simulink library "PCMULib"  (R2022b)
settings: Solver=ode45  StartTime=0.0  StopTime=10.0  RelTol=1e-3  EnableMultiTasking=on
undefined symbols (not defined in the file or in its folder): BreakpointData, BreakpointData1, BreakpointData2, BreakpointData_One_A, BreakpointData_Two_A, caaaa_dbi, caaaa_swi, cTmComprCtrl_n_i16SM4CmpHeatKiMax, cTmComprCtrl_n_i16SM4CmpHeatKiMin, cTmComprCtrl_n_i16SM4CmpHeatKpMax, cTmComprCtrl_n_i16SM4CmpHeatKpMin, cTmComprCtrl_Te_s32ErrCmpPIContinueHeatH, cTmComprCtrl_Te_s32ErrCmpPIContinueHeatL, cTmIn_n_ElacCmprReq_db, cTmIn_n_ElacCmprReq_sw, db, dbi, E2E_P01DataIDMode, E2E_P01ReceiverStatusType, EnumClass, iBit, initalValue, No_Runnable_Period, ObB_EidBsgStDerat_C, p_OVERRIDE_MASTER_SWITCH, SlDemoSign, sw, swi, SwitchOff_P, SwitchOn_P, Table, TableData_M, VCCTi33, VSysD_FidVehDerat1_C
libraries: simulink x22, CCMLib x11, simulink_need_slupdate x9, UXFD_Lib x7, canmsglib x2, PTCC_Lib x1, hdlsllib x1
(part 6 of 7)

== system PCMULib/Standard/Discrete dynamics/LPF1_discreteReset ==
  u : Inport
  a : Inport  Port=2
  r : Inport  Port=3
  LogicalSwitch1 : Subsystem  mask(PAG_Switch_LV1.6_BV2){}
      mask help:
      | Pass through input 1 when input 3 is true;
      | otherwise, pass through input 2
      mask Display:
      | plot([-0.1 0.2 0.2], [0.85 0.85 0.75])
      | plot([-0.1 0.2 0.2], [0.5 0.5 0.6])
      | plot([0.8 1.1], [0.5 0.5])
      | plot([0.15 0.8], [0.6 0.5])
      | plot([-0.1 0.5 0.5], [0.15 0.15 0.6])
  Product : Product  InputSameDT=on  RndMeth=Zero  SaturateOnIntegerOverflow=on  OutDataTypeStr=Inherit: Same as first input  mask(TL_Product){data={'logdata',{'maxnumvals',4096,'plotchannels',[]},'output',{'type','Float32'},'date',735300.29228090274}}
      settings: CopyFcn=if exist('tl_reset_reviewflag','file')==2,tl_reset_reviewflag(gcbh);end  DeleteFcn=if exist('delete_tlblock','file')==2,delete_tlblock(gcbh);end  NameChangeFcn=if exist('rename_tlblock','file')==2,rename_tlblock(gcbh);end  OpenFcn=if exist('tl_open_blockdlg','file')==2,tl_open_blockdlg(gcbh);else,open_system(gcbh,'parameter');end
      mask Help: eval(['if exist(''tl_online_help'',''file'') == 2, tl_online_help(''Topic'',''TL_Product''),else, web([''jar:file:///'',matlabroot,''/help/toolbox/simulink/help.jar!/slref/' lower(get_param(gcbh,'Blocktype')) '.html''], ''-helpbrowser''),end'])
      mask Display: plot([-0.05, 1.05, NaN, -0.05, 1.05],[.01, .01, NaN, .99, .99])
  Sum : Sum  Inputs=+-  InputSameDT=on  SaturateOnIntegerOverflow=on  OutDataTypeStr=Inherit: Same as first input  mask(TL_Sum){data={'logdata',{'maxnumvals',4096,'plotchannels',[]},'output',{'type','Float32'},'date',735300.29228062497}}
      settings: CopyFcn=if exist('tl_reset_reviewflag','file')==2,tl_reset_reviewflag(gcbh);end  DeleteFcn=if exist('delete_tlblock','file')==2,delete_tlblock(gcbh);end  NameChangeFcn=if exist('rename_tlblock','file')==2,rename_tlblock(gcbh);end  OpenFcn=if exist('tl_open_blockdlg','file')==2,tl_open_blockdlg(gcbh);else,open_system(gcbh,'parameter');end
      mask Help: eval(['if exist(''tl_online_help'',''file'') == 2, tl_online_help(''Topic'',''TL_Sum''),else, web([''jar:file:///'',matlabroot,''/help/toolbox/simulink/help.jar!/slref/' lower(get_param(gcbh,'Blocktype')) '.html''], ''-helpbrowser''),end'])
      mask Display: plot([-0.05, 1.05, NaN, -0.05, 1.05],[.01, .01, NaN, .99, .99])
  Sum1 : Sum  InputSameDT=on  SaturateOnIntegerOverflow=on  OutDataTypeStr=Inherit: Same as first input  mask(TL_Sum){data={'logdata',{'maxnumvals',4096,'plotchannels',[]},'output',{'type','Float32'},'date',735300.2922803472}}
      settings: CopyFcn=if exist('tl_reset_reviewflag','file')==2,tl_reset_reviewflag(gcbh);end  DeleteFcn=if exist('delete_tlblock','file')==2,delete_tlblock(gcbh);end  NameChangeFcn=if exist('rename_tlblock','file')==2,rename_tlblock(gcbh);end  OpenFcn=if exist('tl_open_blockdlg','file')==2,tl_open_blockdlg(gcbh);else,open_system(gcbh,'parameter');end
      mask Help: eval(['if exist(''tl_online_help'',''file'') == 2, tl_online_help(''Topic'',''TL_Sum''),else, web([''jar:file:///'',matlabroot,''/help/toolbox/simulink/help.jar!/slref/' lower(get_param(gcbh,'Blocktype')) '.html''], ''-helpbrowser''),end'])
      mask Display: plot([-0.05, 1.05, NaN, -0.05, 1.05],[.01, .01, NaN, .99, .99])
  UnitDelay : UnitDelay  SampleTime=-1  HasFrameUpgradeWarning=on  mask(TL_UnitDelay){data={'logdata',{'maxnumvals',4096,'plotchannels',[]},'output',{'type','Float32'},'state',{'type','Float32'},'date',735300.29228006944}}
      settings: CopyFcn=if exist('tl_reset_reviewflag','file')==2,tl_reset_reviewflag(gcbh);end  DeleteFcn=if exist('delete_tlblock','file')==2,delete_tlblock(gcbh);end  NameChangeFcn=if exist('rename_tlblock','file')==2,rename_tlblock(gcbh);end  OpenFcn=if exist('tl_open_blockdlg','file')==2,tl_open_blockdlg(gcbh);else,open_system(gcbh,'parameter');end
      mask Help: eval(['if exist(''tl_online_help'',''file'') == 2, tl_online_help(''Topic'',''TL_UnitDelay''),else, web([''jar:file:///'',matlabroot,''/help/toolbox/simulink/help.jar!/slref/' lower(get_param(gcbh,'Blocktype')) '.html''], ''-helpbrowser''),end'])
      mask Display: plot([-0.05, 1.05, NaN, -0.05, 1.05],[.01, .01, NaN, .99, .99])
  y : Outport
  wires:
  Product/1 -> Sum1/1
  a/1 -> Product/2
  Sum/1 -> Product/1
  u/1 -> Sum/2, Sum1/2, LogicalSwitch1/1(In1)
  r/1 -> LogicalSwitch1/3(In2)
  UnitDelay/1 -> Sum/1
  Sum1/1 -> LogicalSwitch1/2(In3)
  LogicalSwitch1/1(Out1) -> y/1, UnitDelay/1

== system PCMULib/Standard/Discrete dynamics/LPF2_discrete ==
  u : Inport
  a1 : Inport  Port=2
  a2 : Inport  Port=3
  b0 : Inport  Port=4
  b1 : Inport  Port=5
  b2 : Inport  Port=6
  Product : Product  InputSameDT=on  RndMeth=Zero  SaturateOnIntegerOverflow=on  OutDataTypeStr=Inherit: Same as first input  mask(TL_Product){data={'logdata',{'maxnumvals',4096,'plotchannels',[]},'output',{'type','Float32'},'date',735300.29227971064}}
      settings: CopyFcn=if exist('tl_reset_reviewflag','file')==2,tl_reset_reviewflag(gcbh);end  DeleteFcn=if exist('delete_tlblock','file')==2,delete_tlblock(gcbh);end  NameChangeFcn=if exist('rename_tlblock','file')==2,rename_tlblock(gcbh);end  OpenFcn=if exist('tl_open_blockdlg','file')==2,tl_open_blockdlg(gcbh);else,open_system(gcbh,'parameter');end
      mask Help: eval(['if exist(''tl_online_help'',''file'') == 2, tl_online_help(''Topic'',''TL_Product''),else, web([''jar:file:///'',matlabroot,''/help/toolbox/simulink/help.jar!/slref/' lower(get_param(gcbh,'Blocktype')) '.html''], ''-helpbrowser''),end'])
      mask Display: plot([-0.05, 1.05, NaN, -0.05, 1.05],[.01, .01, NaN, .99, .99])
  Product1 : Product  InputSameDT=on  RndMeth=Zero  SaturateOnIntegerOverflow=on  OutDataTypeStr=Inherit: Same as first input  mask(TL_Product){data={'logdata',{'maxnumvals',4096,'plotchannels',[]},'output',{'type','Float32'},'date',735300.29227943288}}
      settings: CopyFcn=if exist('tl_reset_reviewflag','file')==2,tl_reset_reviewflag(gcbh);end  DeleteFcn=if exist('delete_tlblock','file')==2,delete_tlblock(gcbh);end  NameChangeFcn=if exist('rename_tlblock','file')==2,rename_tlblock(gcbh);end  OpenFcn=if exist('tl_open_blockdlg','file')==2,tl_open_blockdlg(gcbh);else,open_system(gcbh,'parameter');end
      mask Help: eval(['if exist(''tl_online_help'',''file'') == 2, tl_online_help(''Topic'',''TL_Product''),else, web([''jar:file:///'',matlabroot,''/help/toolbox/simulink/help.jar!/slref/' lower(get_param(gcbh,'Blocktype')) '.html''], ''-helpbrowser''),end'])
      mask Display: plot([-0.05, 1.05, NaN, -0.05, 1.05],[.01, .01, NaN, .99, .99])
  Product2 : Product  InputSameDT=on  RndMeth=Zero  SaturateOnIntegerOverflow=on  OutDataTypeStr=Inherit: Same as first input  mask(TL_Product){data={'logdata',{'maxnumvals',4096,'plotchannels',[]},'output',{'type','Float32'},'date',735300.29227915511}}
      settings: CopyFcn=if exist('tl_reset_reviewflag','file')==2,tl_reset_reviewflag(gcbh);end  DeleteFcn=if exist('delete_tlblock','file')==2,delete_tlblock(gcbh);end  NameChangeFcn=if exist('rename_tlblock','file')==2,rename_tlblock(gcbh);end  OpenFcn=if exist('tl_open_blockdlg','file')==2,tl_open_blockdlg(gcbh);else,open_system(gcbh,'parameter');end
      mask Help: eval(['if exist(''tl_online_help'',''file'') == 2, tl_online_help(''Topic'',''TL_Product''),else, web([''jar:file:///'',matlabroot,''/help/toolbox/simulink/help.jar!/slref/' lower(get_param(gcbh,'Blocktype')) '.html''], ''-helpbrowser''),end'])
      mask Display: plot([-0.05, 1.05, NaN, -0.05, 1.05],[.01, .01, NaN, .99, .99])
  Product3 : Product  InputSameDT=on  RndMeth=Zero  SaturateOnIntegerOverflow=on  OutDataTypeStr=Inherit: Same as first input  mask(TL_Product){data={'logdata',{'maxnumvals',4096,'plotchannels',[]},'output',{'type','Float32'},'date',735300.29227888887}}
      settings: CopyFcn=if exist('tl_reset_reviewflag','file')==2,tl_reset_reviewflag(gcbh);end  DeleteFcn=if exist('delete_tlblock','file')==2,delete_tlblock(gcbh);end  NameChangeFcn=if exist('rename_tlblock','file')==2,rename_tlblock(gcbh);end  OpenFcn=if exist('tl_open_blockdlg','file')==2,tl_open_blockdlg(gcbh);else,open_system(gcbh,'parameter');end
      mask Help: eval(['if exist(''tl_online_help'',''file'') == 2, tl_online_help(''Topic'',''TL_Product''),else, web([''jar:file:///'',matlabroot,''/help/toolbox/simulink/help.jar!/slref/' lower(get_param(gcbh,'Blocktype')) '.html''], ''-helpbrowser''),end'])
      mask Display: plot([-0.05, 1.05, NaN, -0.05, 1.05],[.01, .01, NaN, .99, .99])
  Product4 : Product  InputSameDT=on  RndMeth=Zero  SaturateOnIntegerOverflow=on  OutDataTypeStr=Inherit: Same as first input  mask(TL_Product){data={'logdata',{'maxnumvals',4096,'plotchannels',[]},'output',{'type','Float32'},'date',735300.2922786111}}
      settings: CopyFcn=if exist('tl_reset_reviewflag','file')==2,tl_reset_reviewflag(gcbh);end  DeleteFcn=if exist('delete_tlblock','file')==2,delete_tlblock(gcbh);end  NameChangeFcn=if exist('rename_tlblock','file')==2,rename_tlblock(gcbh);end  OpenFcn=if exist('tl_open_blockdlg','file')==2,tl_open_blockdlg(gcbh);else,open_system(gcbh,'parameter');end
      mask Help: eval(['if exist(''tl_online_help'',''file'') == 2, tl_online_help(''Topic'',''TL_Product''),else, web([''jar:file:///'',matlabroot,''/help/toolbox/simulink/help.jar!/slref/' lower(get_param(gcbh,'Blocktype')) '.html''], ''-helpbrowser''),end'])
      mask Display: plot([-0.05, 1.05, NaN, -0.05, 1.05],[.01, .01, NaN, .99, .99])
  Sum : Sum  Inputs=+++--  InputSameDT=on  SaturateOnIntegerOverflow=on  OutDataTypeStr=Inherit: Same as first input  mask(TL_Sum){data={'logdata',{'maxnumvals',4096,'plotchannels',[]},'output',{'type','Float32'},'date',735300.29227833333}}
      settings: CopyFcn=if exist('tl_reset_reviewflag','file')==2,tl_reset_reviewflag(gcbh);end  DeleteFcn=if exist('delete_tlblock','file')==2,delete_tlblock(gcbh);end  NameChangeFcn=if exist('rename_tlblock','file')==2,rename_tlblock(gcbh);end  OpenFcn=if exist('tl_open_blockdlg','file')==2,tl_open_blockdlg(gcbh);else,open_system(gcbh,'parameter');end
      mask Help: eval(['if exist(''tl_online_help'',''file'') == 2, tl_online_help(''Topic'',''TL_Sum''),else, web([''jar:file:///'',matlabroot,''/help/toolbox/simulink/help.jar!/slref/' lower(get_param(gcbh,'Blocktype')) '.html''], ''-helpbrowser''),end'])
      mask Display: plot([-0.05, 1.05, NaN, -0.05, 1.05],[.01, .01, NaN, .99, .99])
  UnitDelay : UnitDelay  SampleTime=-1  HasFrameUpgradeWarning=on  mask(TL_UnitDelay){data={'logdata',{'maxnumvals',4096,'plotchannels',[]},'output',{'type','Float32'},'state',{'type','Float32'},'date',735300.29227804393}}
      settings: CopyFcn=if exist('tl_reset_reviewflag','file')==2,tl_reset_reviewflag(gcbh);end  DeleteFcn=if exist('delete_tlblock','file')==2,delete_tlblock(gcbh);end  NameChangeFcn=if exist('rename_tlblock','file')==2,rename_tlblock(gcbh);end  OpenFcn=if exist('tl_open_blockdlg','file')==2,tl_open_blockdlg(gcbh);else,open_system(gcbh,'parameter');end
      mask Help: eval(['if exist(''tl_online_help'',''file'') == 2, tl_online_help(''Topic'',''TL_UnitDelay''),else, web([''jar:file:///'',matlabroot,''/help/toolbox/simulink/help.jar!/slref/' lower(get_param(gcbh,'Blocktype')) '.html''], ''-helpbrowser''),end'])
      mask Display: plot([-0.05, 1.05, NaN, -0.05, 1.05],[.01, .01, NaN, .99, .99])
  UnitDelay1 : UnitDelay  SampleTime=-1  HasFrameUpgradeWarning=on  mask(TL_UnitDelay){data={'logdata',{'maxnumvals',4096,'plotchannels',[]},'output',{'type','Float32'},'state',{'type','Float32'},'date',735300.29227769678}}
      settings: CopyFcn=if exist('tl_reset_reviewflag','file')==2,tl_reset_reviewflag(gcbh);end  DeleteFcn=if exist('delete_tlblock','file')==2,delete_tlblock(gcbh);end  NameChangeFcn=if exist('rename_tlblock','file')==2,rename_tlblock(gcbh);end  OpenFcn=if exist('tl_open_blockdlg','file')==2,tl_open_blockdlg(gcbh);else,open_system(gcbh,'parameter');end
      mask Help: eval(['if exist(''tl_online_help'',''file'') == 2, tl_online_help(''Topic'',''TL_UnitDelay''),else, web([''jar:file:///'',matlabroot,''/help/toolbox/simulink/help.jar!/slref/' lower(get_param(gcbh,'Blocktype')) '.html''], ''-helpbrowser''),end'])
      mask Display: plot([-0.05, 1.05, NaN, -0.05, 1.05],[.01, .01, NaN, .99, .99])
  UnitDelay2 : UnitDelay  SampleTime=-1  HasFrameUpgradeWarning=on  mask(TL_UnitDelay){data={'logdata',{'maxnumvals',4096,'plotchannels',[]},'output',{'type','Float32'},'state',{'type','Float32'},'date',735300.29227733798}}
      settings: CopyFcn=if exist('tl_reset_reviewflag','file')==2,tl_reset_reviewflag(gcbh);end  DeleteFcn=if exist('delete_tlblock','file')==2,delete_tlblock(gcbh);end  NameChangeFcn=if exist('rename_tlblock','file')==2,rename_tlblock(gcbh);end  OpenFcn=if exist('tl_open_blockdlg','file')==2,tl_open_blockdlg(gcbh);else,open_system(gcbh,'parameter');end
      mask Help: eval(['if exist(''tl_online_help'',''file'') == 2, tl_online_help(''Topic'',''TL_UnitDelay''),else, web([''jar:file:///'',matlabroot,''/help/toolbox/simulink/help.jar!/slref/' lower(get_param(gcbh,'Blocktype')) '.html''], ''-helpbrowser''),end'])
      mask Display: plot([-0.05, 1.05, NaN, -0.05, 1.05],[.01, .01, NaN, .99, .99])
  UnitDelay3 : UnitDelay  SampleTime=-1  HasFrameUpgradeWarning=on  mask(TL_UnitDelay){data={'logdata',{'maxnumvals',4096,'plotchannels',[]},'output',{'type','Float32'},'state',{'type','Float32'},'date',735300.29227697919}}
      settings: CopyFcn=if exist('tl_reset_reviewflag','file')==2,tl_reset_reviewflag(gcbh);end  DeleteFcn=if exist('delete_tlblock','file')==2,delete_tlblock(gcbh);end  NameChangeFcn=if exist('rename_tlblock','file')==2,rename_tlblock(gcbh);end  OpenFcn=if exist('tl_open_blockdlg','file')==2,tl_open_blockdlg(gcbh);else,open_system(gcbh,'parameter');end
      mask Help: eval(['if exist(''tl_online_help'',''file'') == 2, tl_online_help(''Topic'',''TL_UnitDelay''),else, web([''jar:file:///'',matlabroot,''/help/toolbox/simulink/help.jar!/slref/' lower(get_param(gcbh,'Blocktype')) '.html''], ''-helpbrowser''),end'])
      mask Display: plot([-0.05, 1.05, NaN, -0.05, 1.05],[.01, .01, NaN, .99, .99])
  y : Outport
  wires:
  UnitDelay3/1 -> Product4/2
  Product2/1 -> Sum/1
  Product1/1 -> Sum/2
  UnitDelay2/1 -> Product2/1
  b2/1 -> Product2/2
  b1/1 -> Product1/2
  Product/1 -> Sum/3
  Product3/1 -> Sum/4
  a1/1 -> Product3/1
  b0/1 -> Product/2
  a2/1 -> Product4/1
  Product4/1 -> Sum/5
  UnitDelay/1 -> UnitDelay2/1, Product1/1
  u/1 -> UnitDelay/1, Product/1
  Sum/1 -> y/1, UnitDelay1/1
  UnitDelay1/1 -> Product3/2, UnitDelay3/1

== system PCMULib/Standard/Discrete dynamics/LPF2_omega ==
  u : Inport
  w : Inport  Port=2
  z : Inport  Port=3
  Constant : Constant  Value=2  mask(TL_Constant){data={'output',{'type','Float32'},'date',735300.29222866893}}
      settings: CopyFcn=if exist('tl_reset_reviewflag','file')==2,tl_reset_reviewflag(gcbh);end  DeleteFcn=if exist('delete_tlblock','file')==2,delete_tlblock(gcbh);end  NameChangeFcn=if exist('rename_tlblock','file')==2,rename_tlblock(gcbh);end  OpenFcn=if exist('tl_open_blockdlg','file')==2,tl_open_blockdlg(gcbh);else,open_system(gcbh,'parameter');end
      mask Help: eval(['if exist(''tl_online_help'',''file'') == 2, tl_online_help(''Topic'',''TL_Constant''),else, web([''jar:file:///'',matlabroot,''/help/toolbox/simulink/help.jar!/slref/' lower(get_param(gcbh,'Blocktype')) '.html''], ''-helpbrowser''),end'])
      mask Display: plot([-0.05, 1.05, NaN, -0.05, 1.05],[.01, .01, NaN, .99, .99])
  Constant2 : Constant  Value=2  mask(TL_Constant){data={'output',{'type','Float32'},'date',735300.29222841433}}
      settings: CopyFcn=if exist('tl_reset_reviewflag','file')==2,tl_reset_reviewflag(gcbh);end  DeleteFcn=if exist('delete_tlblock','file')==2,delete_tlblock(gcbh);end  NameChangeFcn=if exist('rename_tlblock','file')==2,rename_tlblock(gcbh);end  OpenFcn=if exist('tl_open_blockdlg','file')==2,tl_open_blockdlg(gcbh);else,open_system(gcbh,'parameter');end
      mask Help: eval(['if exist(''tl_online_help'',''file'') == 2, tl_online_help(''Topic'',''TL_Constant''),else, web([''jar:file:///'',matlabroot,''/help/toolbox/simulink/help.jar!/slref/' lower(get_param(gcbh,'Blocktype')) '.html''], ''-helpbrowser''),end'])
      mask Display: plot([-0.05, 1.05, NaN, -0.05, 1.05],[.01, .01, NaN, .99, .99])
  Constant3 : Constant  mask(TL_Constant){data={'output',{'type','Float32'},'date',735300.29222815973}}
      settings: CopyFcn=if exist('tl_reset_reviewflag','file')==2,tl_reset_reviewflag(gcbh);end  DeleteFcn=if exist('delete_tlblock','file')==2,delete_tlblock(gcbh);end  NameChangeFcn=if exist('rename_tlblock','file')==2,rename_tlblock(gcbh);end  OpenFcn=if exist('tl_open_blockdlg','file')==2,tl_open_blockdlg(gcbh);else,open_system(gcbh,'parameter');end
      mask Help: eval(['if exist(''tl_online_help'',''file'') == 2, tl_online_help(''Topic'',''TL_Constant''),else, web([''jar:file:///'',matlabroot,''/help/toolbox/simulink/help.jar!/slref/' lower(get_param(gcbh,'Blocktype')) '.html''], ''-helpbrowser''),end'])
      mask Display: plot([-0.05, 1.05, NaN, -0.05, 1.05],[.01, .01, NaN, .99, .99])
  Product : Product  Inputs=**  InputSameDT=on  RndMeth=Zero  SaturateOnIntegerOverflow=on  OutDataTypeStr=Inherit: Same as first input  mask(TL_Product){data={'logdata',{'maxnumvals',4096,'plotchannels',[]},'output',{'type','Float32'},'date',735300.29222787032}}
      settings: CopyFcn=if exist('tl_reset_reviewflag','file')==2,tl_reset_reviewflag(gcbh);end  DeleteFcn=if exist('delete_tlblock','file')==2,delete_tlblock(gcbh);end  NameChangeFcn=if exist('rename_tlblock','file')==2,rename_tlblock(gcbh);end  OpenFcn=if exist('tl_open_blockdlg','file')==2,tl_open_blockdlg(gcbh);else,open_system(gcbh,'parameter');end
      mask Help: eval(['if exist(''tl_online_help'',''file'') == 2, tl_online_help(''Topic'',''TL_Product''),else, web([''jar:file:///'',matlabroot,''/help/toolbox/simulink/help.jar!/slref/' lower(get_param(gcbh,'Blocktype')) '.html''], ''-helpbrowser''),end'])
      mask Display: plot([-0.05, 1.05, NaN, -0.05, 1.05],[.01, .01, NaN, .99, .99])
  Product1 : Product  Inputs=***  InputSameDT=on  RndMeth=Zero  SaturateOnIntegerOverflow=on  OutDataTypeStr=Inherit: Same as first input  mask(TL_Product){data={'logdata',{'maxnumvals',4096,'plotchannels',[]},'output',{'type','Float32'},'date',735300.29222759255}}
      settings: CopyFcn=if exist('tl_reset_reviewflag','file')==2,tl_reset_reviewflag(gcbh);end  DeleteFcn=if exist('delete_tlblock','file')==2,delete_tlblock(gcbh);end  NameChangeFcn=if exist('rename_tlblock','file')==2,rename_tlblock(gcbh);end  OpenFcn=if exist('tl_open_blockdlg','file')==2,tl_open_blockdlg(gcbh);else,open_system(gcbh,'parameter');end
      mask Help: eval(['if exist(''tl_online_help'',''file'') == 2, tl_online_help(''Topic'',''TL_Product''),else, web([''jar:file:///'',matlabroot,''/help/toolbox/simulink/help.jar!/slref/' lower(get_param(gcbh,'Blocktype')) '.html''], ''-helpbrowser''),end'])
      mask Display: plot([-0.05, 1.05, NaN, -0.05, 1.05],[.01, .01, NaN, .99, .99])
  Product3 : Product  Inputs=**  InputSameDT=on  RndMeth=Zero  SaturateOnIntegerOverflow=on  OutDataTypeStr=Inherit: Same as first input  mask(TL_Product){data={'logdata',{'maxnumvals',4096,'plotchannels',[]},'output',{'type','Float32'},'date',735300.29222732643}}
      settings: CopyFcn=if exist('tl_reset_reviewflag','file')==2,tl_reset_reviewflag(gcbh);end  DeleteFcn=if exist('delete_tlblock','file')==2,delete_tlblock(gcbh);end  NameChangeFcn=if exist('rename_tlblock','file')==2,rename_tlblock(gcbh);end  OpenFcn=if exist('tl_open_blockdlg','file')==2,tl_open_blockdlg(gcbh);else,open_system(gcbh,'parameter');end
      mask Help: eval(['if exist(''tl_online_help'',''file'') == 2, tl_online_help(''Topic'',''TL_Product''),else, web([''jar:file:///'',matlabroot,''/help/toolbox/simulink/help.jar!/slref/' lower(get_param(gcbh,'Blocktype')) '.html''], ''-helpbrowser''),end'])
      mask Display: plot([-0.05, 1.05, NaN, -0.05, 1.05],[.01, .01, NaN, .99, .99])
  Product4 : Product  Inputs=**  InputSameDT=on  RndMeth=Zero  SaturateOnIntegerOverflow=on  OutDataTypeStr=Inherit: Same as first input  mask(TL_Product){data={'logdata',{'maxnumvals',4096,'plotchannels',[]},'output',{'type','Float32'},'date',735300.29222704866}}
      settings: CopyFcn=if exist('tl_reset_reviewflag','file')==2,tl_reset_reviewflag(gcbh);end  DeleteFcn=if exist('delete_tlblock','file')==2,delete_tlblock(gcbh);end  NameChangeFcn=if exist('rename_tlblock','file')==2,rename_tlblock(gcbh);end  OpenFcn=if exist('tl_open_blockdlg','file')==2,tl_open_blockdlg(gcbh);else,open_system(gcbh,'parameter');end
      mask Help: eval(['if exist(''tl_online_help'',''file'') == 2, tl_online_help(''Topic'',''TL_Product''),else, web([''jar:file:///'',matlabroot,''/help/toolbox/simulink/help.jar!/slref/' lower(get_param(gcbh,'Blocktype')) '.html''], ''-helpbrowser''),end'])
      mask Display: plot([-0.05, 1.05, NaN, -0.05, 1.05],[.01, .01, NaN, .99, .99])
  Product5 : Product  Inputs=*/  InputSameDT=on  RndMeth=Zero  SaturateOnIntegerOverflow=on  OutDataTypeStr=Inherit: Same as first input  mask(TL_Product){data={'logdata',{'maxnumvals',4096,'plotchannels',[]},'output',{'type','Float32'},'date',735300.29222677078}}
      settings: CopyFcn=if exist('tl_reset_reviewflag','file')==2,tl_reset_reviewflag(gcbh);end  DeleteFcn=if exist('delete_tlblock','file')==2,delete_tlblock(gcbh);end  NameChangeFcn=if exist('rename_tlblock','file')==2,rename_tlblock(gcbh);end  OpenFcn=if exist('tl_open_blockdlg','file')==2,tl_open_blockdlg(gcbh);else,open_system(gcbh,'parameter');end
      mask Help: eval(['if exist(''tl_online_help'',''file'') == 2, tl_online_help(''Topic'',''TL_Product''),else, web([''jar:file:///'',matlabroot,''/help/toolbox/simulink/help.jar!/slref/' lower(get_param(gcbh,'Blocktype')) '.html''], ''-helpbrowser''),end'])
      mask Display: plot([-0.05, 1.05, NaN, -0.05, 1.05],[.01, .01, NaN, .99, .99])
  Product6 : Product  Inputs=**  InputSameDT=on  RndMeth=Zero  SaturateOnIntegerOverflow=on  OutDataTypeStr=Inherit: Same as first input  mask(TL_Product){data={'logdata',{'maxnumvals',4096,'plotchannels',[]},'output',{'type','Float32'},'date',735300.29222649301}}
      settings: CopyFcn=if exist('tl_reset_reviewflag','file')==2,tl_reset_reviewflag(gcbh);end  DeleteFcn=if exist('delete_tlblock','file')==2,delete_tlblock(gcbh);end  NameChangeFcn=if exist('rename_tlblock','file')==2,rename_tlblock(gcbh);end  OpenFcn=if exist('tl_open_blockdlg','file')==2,tl_open_blockdlg(gcbh);else,open_system(gcbh,'parameter');end
      mask Help: eval(['if exist(''tl_online_help'',''file'') == 2, tl_online_help(''Topic'',''TL_Product''),else, web([''jar:file:///'',matlabroot,''/help/toolbox/simulink/help.jar!/slref/' lower(get_param(gcbh,'Blocktype')) '.html''], ''-helpbrowser''),end'])
      mask Display: plot([-0.05, 1.05, NaN, -0.05, 1.05],[.01, .01, NaN, .99, .99])
  Sum1 : Sum  Inputs=+--  InputSameDT=on  SaturateOnIntegerOverflow=on  OutDataTypeStr=Inherit: Same as first input  mask(TL_Sum){data={'logdata',{'maxnumvals',4096,'plotchannels',[]},'output',{'type','Float32'},'date',735300.29222619208}}
      settings: CopyFcn=if exist('tl_reset_reviewflag','file')==2,tl_reset_reviewflag(gcbh);end  DeleteFcn=if exist('delete_tlblock','file')==2,delete_tlblock(gcbh);end  NameChangeFcn=if exist('rename_tlblock','file')==2,rename_tlblock(gcbh);end  OpenFcn=if exist('tl_open_blockdlg','file')==2,tl_open_blockdlg(gcbh);else,open_system(gcbh,'parameter');end
      mask Help: eval(['if exist(''tl_online_help'',''file'') == 2, tl_online_help(''Topic'',''TL_Sum''),else, web([''jar:file:///'',matlabroot,''/help/toolbox/simulink/help.jar!/slref/' lower(get_param(gcbh,'Blocktype')) '.html''], ''-helpbrowser''),end'])
      mask Display: plot([-0.05, 1.05, NaN, -0.05, 1.05],[.01, .01, NaN, .99, .99])
  Sum2 : Sum  Inputs=--  InputSameDT=on  SaturateOnIntegerOverflow=on  OutDataTypeStr=Inherit: Same as first input  mask(TL_Sum){data={'logdata',{'maxnumvals',4096,'plotchannels',[]},'output',{'type','Float32'},'date',735300.29222592595}}
      settings: CopyFcn=if exist('tl_reset_reviewflag','file')==2,tl_reset_reviewflag(gcbh);end  DeleteFcn=if exist('delete_tlblock','file')==2,delete_tlblock(gcbh);end  NameChangeFcn=if exist('rename_tlblock','file')==2,rename_tlblock(gcbh);end  OpenFcn=if exist('tl_open_blockdlg','file')==2,tl_open_blockdlg(gcbh);else,open_system(gcbh,'parameter');end
      mask Help: eval(['if exist(''tl_online_help'',''file'') == 2, tl_online_help(''Topic'',''TL_Sum''),else, web([''jar:file:///'',matlabroot,''/help/toolbox/simulink/help.jar!/slref/' lower(get_param(gcbh,'Blocktype')) '.html''], ''-helpbrowser''),end'])
      mask Display: plot([-0.05, 1.05, NaN, -0.05, 1.05],[.01, .01, NaN, .99, .99])
  Sum3 : Sum  Inputs=+++  InputSameDT=on  SaturateOnIntegerOverflow=on  OutDataTypeStr=Inherit: Same as first input  mask(TL_Sum){data={'logdata',{'maxnumvals',4096,'plotchannels',[]},'output',{'type','Float32'},'date',735300.29222564818}}
      settings: CopyFcn=if exist('tl_reset_reviewflag','file')==2,tl_reset_reviewflag(gcbh);end  DeleteFcn=if exist('delete_tlblock','file')==2,delete_tlblock(gcbh);end  NameChangeFcn=if exist('rename_tlblock','file')==2,rename_tlblock(gcbh);end  OpenFcn=if exist('tl_open_blockdlg','file')==2,tl_open_blockdlg(gcbh);else,open_system(gcbh,'parameter');end
      mask Help: eval(['if exist(''tl_online_help'',''file'') == 2, tl_online_help(''Topic'',''TL_Sum''),else, web([''jar:file:///'',matlabroot,''/help/toolbox/simulink/help.jar!/slref/' lower(get_param(gcbh,'Blocktype')) '.html''], ''-helpbrowser''),end'])
      mask Display: plot([-0.05, 1.05, NaN, -0.05, 1.05],[.01, .01, NaN, .99, .99])
  UnitDelay1 : UnitDelay  SampleTime=-1  HasFrameUpgradeWarning=on  mask(TL_UnitDelay){data={'logdata',{'maxnumvals',4096,'plotchannels',[]},'output',{'type','Float32'},'state',{'type','Float32'},'date',735300.29222532408}}
      settings: CopyFcn=if exist('tl_reset_reviewflag','file')==2,tl_reset_reviewflag(gcbh);end  DeleteFcn=if exist('delete_tlblock','file')==2,delete_tlblock(gcbh);end  NameChangeFcn=if exist('rename_tlblock','file')==2,rename_tlblock(gcbh);end  OpenFcn=if exist('tl_open_blockdlg','file')==2,tl_open_blockdlg(gcbh);else,open_system(gcbh,'parameter');end
      mask Help: eval(['if exist(''tl_online_help'',''file'') == 2, tl_online_help(''Topic'',''TL_UnitDelay''),else, web([''jar:file:///'',matlabroot,''/help/toolbox/simulink/help.jar!/slref/' lower(get_param(gcbh,'Blocktype')) '.html''], ''-helpbrowser''),end'])
      mask Display: plot([-0.05, 1.05, NaN, -0.05, 1.05],[.01, .01, NaN, .99, .99])
  UnitDelay3 : UnitDelay  SampleTime=-1  HasFrameUpgradeWarning=on  mask(TL_UnitDelay){data={'logdata',{'maxnumvals',4096,'plotchannels',[]},'output',{'type','Float32'},'state',{'type','Float32'},'date',735300.29222478007}}
      settings: CopyFcn=if exist('tl_reset_reviewflag','file')==2,tl_reset_reviewflag(gcbh);end  DeleteFcn=if exist('delete_tlblock','file')==2,delete_tlblock(gcbh);end  NameChangeFcn=if exist('rename_tlblock','file')==2,rename_tlblock(gcbh);end  OpenFcn=if exist('tl_open_blockdlg','file')==2,tl_open_blockdlg(gcbh);else,open_system(gcbh,'parameter');end
      mask Help: eval(['if exist(''tl_online_help'',''file'') == 2, tl_online_help(''Topic'',''TL_UnitDelay''),else, web([''jar:file:///'',matlabroot,''/help/toolbox/simulink/help.jar!/slref/' lower(get_param(gcbh,'Blocktype')) '.html''], ''-helpbrowser''),end'])
      mask Display: plot([-0.05, 1.05, NaN, -0.05, 1.05],[.01, .01, NaN, .99, .99])
  ts : DataStoreRead  DataStoreName=ts  IndexOptions=Index vector (dialog)  Indices=1  OutputSizes=1  mask(TL_DataStoreRead){data={'logdata',{'plotchannels',[]},'date',735300.29222303245}}
      settings: AttributesFormatString=ts  DeleteFcn=if exist('delete_tlblock','file')==2,delete_tlblock(gcbh);end  NameChangeFcn=if exist('rename_tlblock','file')==2,rename_tlblock(gcbh);end  OpenFcn=if exist('tl_open_blockdlg','file')==2,tl_open_blockdlg(gcbh);else,open_system(gcbh,'parameter');end
      mask Help: eval(['if exist(''tl_online_help'',''file'') == 2, tl_online_help(''Topic'',''TL_DataStoreRead''),else, web([''jar:file:///'',matlabroot,''/help/toolbox/simulink/help.jar!/slref/' lower(get_param(gcbh,'Blocktype')) '.html''], ''-helpbrowser''),end'])
      mask Display: plot([-0.05, 1.05, NaN, -0.05, 1.05],[.01, .01, NaN, .99, .99])
  y : Outport
  wires:
  z/1 -> Product1/2
  UnitDelay3/1 -> Sum1/3
  Product3/1 -> Product6/2, Sum3/2
  Sum3/1 -> Product5/2
  Constant3/1 -> Sum3/3
  Product5/1 -> y/1, UnitDelay1/1
  Constant2/1 -> Sum2/1
  u/1 -> Product6/1
  Product6/1 -> Sum1/1
  Product4/1 -> Sum1/2
  Sum1/1 -> Product5/1
  Sum2/1 -> Product4/1
  ts/1 -> Product/2
  w/1 -> Product/1
  Constant/1 -> Product1/3
  Product1/1 -> Sum3/1, Sum2/2
  UnitDelay1/1 -> Product4/2, UnitDelay3/1
  Product/1 -> Product1/1, Product3/2, Product3/1

== system PCMULib/Standard/Discrete dynamics/RateLimit ==
  u : Inport
  d : Inport  Port=2
  Add : Sum  Inputs=+-
  Add1 : Sum
  MinMax : MinMax  Function=max  Inputs=2
  MinMax1 : MinMax  Inputs=2
  Product : Product
  Product1 : Product
  Unit Delay : UnitDelay  SampleTime=-1  HasFrameUpgradeWarning=on
  ts : DataStoreRead  DataStoreName=ts  IndexOptions=Index vector (dialog)  Indices=1  OutputSizes=1
  y : Outport
  wires:
  d/1 -> Product/1, Product1/2
  Product/1 -> Add1/1
  ts/1 -> Product/2, Product1/1
  Product1/1 -> Add/2
  Add/1 -> MinMax/2
  MinMax/1 -> MinMax1/1
  Unit Delay/1 -> Add1/2, Add/1
  Add1/1 -> MinMax1/2
  u/1 -> MinMax/1
  MinMax1/1 -> y/1, Unit Delay/1

== system PCMULib/Standard/Discrete dynamics/RateLimit1 ==
  In1 : Inport
  r : Inport  Port=2
  dr : Inport  Port=3
  r1 : Inport  Port=4
  Abs : Abs  SaturateOnIntegerOverflow=off
  Add : Sum  Inputs=+-
  Add1 : Sum
  MinMax : MinMax  Function=max  Inputs=2
  MinMax1 : MinMax  Inputs=2
  Product : Product
  Product1 : Product
  Switch : Switch  Criteria=u2 > Threshold  SaturateOnIntegerOverflow=off  InputSameDT=off
  Unit Delay : UnitDelay  SampleTime=-1  HasFrameUpgradeWarning=on
  ts : DataStoreRead  DataStoreName=ts  IndexOptions=Index vector (dialog)  Indices=1  OutputSizes=1
  y : Outport
  wires:
  Abs/1 -> Add/2
  In1/1 -> Switch/1, MinMax/1
  Add1/1 -> MinMax1/2
  Unit Delay/1 -> Add1/2, Add/1
  MinMax/1 -> MinMax1/1
  Product1/1 -> Abs/1
  ts/1 -> Product1/1, Product/2
  Product/1 -> Add1/1
  dr/1 -> Product/1
  MinMax1/1 -> Switch/3
  r/1 -> Switch/2
  Switch/1 -> y/1, Unit Delay/1
  r1/1 -> Product1/2
  Add/1 -> MinMax/2

== system PCMULib/Standard/Discrete dynamics/xbackground1 ==

== system PCMULib/Standard/Discrete dynamics/xbackground2 ==

== system PCMULib/Standard/Discrete dynamics/xbackground3 ==

== system PCMULib/Standard/Discrete dynamics/xbackground4 ==

== system PCMULib/Standard/Discrete dynamics/xbackground5 ==

== system PCMULib/Standard/Discrete dynamics/xbackground6 ==

== system PCMULib/Standard/Discrete dynamics/xbackground7 ==

== system PCMULib/Standard/Math/AbsForBoschCompiler ==
  In1 : Inport
  Gain : Gain  Gain=-1  OutDataTypeStr=Inherit: Same as input  ParamDataTypeStr=Inherit: Same as input  mask(TL_Gain){data={'logdata',{'plotchannels',[]},'output',{'type','Float32','unit','-'},'date',735300.29225025466}}
      settings: CopyFcn=if exist('tl_reset_reviewflag','file')==2,tl_reset_reviewflag(gcbh);end  DeleteFcn=if exist('delete_tlblock','file')==2,delete_tlblock(gcbh);end  NameChangeFcn=if exist('rename_tlblock','file')==2,rename_tlblock(gcbh);end  OpenFcn=if exist('tl_open_blockdlg','file')==2,tl_open_blockdlg(gcbh);else,open_system(gcbh,'parameter');end
      mask Help: eval(['if exist(''tl_online_help'',''file'') == 2, tl_online_help(''Topic'',''TL_Gain''),else, web([''jar:file:///'',matlabroot,''/help/toolbox/simulink/help.jar!/slref/' lower(get_param(gcbh,'Blocktype')) '.html''], ''-helpbrowser''),end'])
      mask Display: plot([0, .9, 0],[.05, .5, .95])
  Switch1 : Switch  SaturateOnIntegerOverflow=off  InputSameDT=off  mask(TL_Switch){data={'logdata',{'plotchannels',[]},'output',{'name','r$N_$L','class','CVC_DISP32','type','Float32'},'date',737070.42928155093}}
      settings: CopyFcn=if exist('tl_reset_reviewflag','file')==2,tl_reset_reviewflag(gcbh);end  DeleteFcn=if exist('delete_tlblock','file')==2,delete_tlblock(gcbh);end  NameChangeFcn=if exist('rename_tlblock','file')==2,rename_tlblock(gcbh);end  OpenFcn=if exist('tl_open_blockdlg','file')==2,tl_open_blockdlg(gcbh);else,open_system(gcbh,'parameter');end
      mask Help: eval(['if exist(''tl_online_help'',''file'') == 2, tl_online_help(''Topic'',''TL_Switch''),else, web([''jar:file:///'',matlabroot,''/help/toolbox/simulink/help.jar!/slref/' lower(get_param(gcbh,'Blocktype')) '.html''], ''-helpbrowser''),end'])
      mask Display: plot([-0.05, 1.05, NaN, -0.05, 1.05],[.01, .01, NaN, .99, .99])
  Out1 : Outport
  wires:
  Gain/1 -> Switch1/3
  In1/1 -> Gain/1, Switch1/2, Switch1/1
  Switch1/1 -> Out1/1  "rt_DFT2RevArgAbs"

== system PCMULib/Standard/Math/Floor ==
  In1 : Inport
  Add : Sum  Inputs=+-
  Constant : Constant
  mod1 : Subsystem  mask(GL_Mod_1.0){}
      mask help: Signed remainder after division.
      mask Display: disp('mod')
  Out1 : Outport
  wires:
  Constant/1 -> mod1/2(In2)
  Add/1 -> Out1/1
  In1/1 -> mod1/1(In1), Add/1
  mod1/1(Out1) -> Add/2

== system PCMULib/Standard/Math/Interpolation ==
  In1 : Inport
  x1 : Inport  Port=2
  y1 : Inport  Port=3
  x2 : Inport  Port=4
  y2 : Inport  Port=5
  Add : Sum  Inputs=+-
  Add1 : Sum  Inputs=+-
  Add2 : Sum  Inputs=+-
  Add3 : Sum
  Constant : Constant
  One3 : Constant  Value=1e-6  OutDataTypeStr=single  mask(TL_Constant){data={'output',{'type','Float32'},'date',735300.29224869213}}
      settings: CopyFcn=if exist('tl_reset_reviewflag','file')==2,tl_reset_reviewflag(gcbh);end  DeleteFcn=if exist('delete_tlblock','file')==2,delete_tlblock(gcbh);end  NameChangeFcn=if exist('rename_tlblock','file')==2,rename_tlblock(gcbh);end  OpenFcn=if exist('tl_open_blockdlg','file')==2,tl_open_blockdlg(gcbh);else,open_system(gcbh,'parameter');end
      mask Help: eval(['if exist(''tl_online_help'',''file'') == 2, tl_online_help(''Topic'',''TL_Constant''),else, web([''jar:file:///'',matlabroot,''/help/toolbox/simulink/help.jar!/slref/' lower(get_param(gcbh,'Blocktype')) '.html''], ''-helpbrowser''),end'])
      mask Display: plot([-0.05, 1.05, NaN, -0.05, 1.05],[.01, .01, NaN, .99, .99])
  Product : Product
  Product1 : Product
  Safe_Divide : Subsystem  mask(GL_SafeDivide_1.0){}
      mask help:
      | Safe Divide, prevents division by zero.
      |
      | if abs(denominator) > eps then
      |     output = numerator / denominator
      | else
      |     output = numerator / eps
      |
      | Attention!
      | Use this block only when there is a risk for division by zero.
      mask init:
      | set_param(gcb,'LinkStatus','none');
      mask Display:
      | port_label('input', 1, 'x')
      | port_label('input', 2, '÷')
      | port_label('input', 3, 'eps')
  Out1 : Outport
  wires:
  In1/1 -> Add/1
  x1/1 -> Add1/2, Add/2
  Add/1 -> Safe_Divide/1(In3)
  Constant/1 -> Add2/1
  Add2/1 -> Product/2
  Product1/1 -> Add3/2
  Product/1 -> Add3/1
  Add1/1 -> Safe_Divide/2(In2)
  Add3/1 -> Out1/1
  y1/1 -> Product/1
  y2/1 -> Product1/2
  Safe_Divide/1(Out1) -> Product1/1, Add2/2
  x2/1 -> Add1/1
  One3/1 -> Safe_Divide/3(In1)

== system PCMULib/Standard/Math/LimitInterpolation ==
  In1 : Inport
  x1 : Inport  Port=2
  y1 : Inport  Port=3
  x2 : Inport  Port=4
  y2 : Inport  Port=5
  Add : Sum  Inputs=+-
  Add1 : Sum  Inputs=+-
  Add2 : Sum  Inputs=+-
  Add3 : Sum
  Constant : Constant
  Constant1 : Constant  Value=0
  Constant2 : Constant
  One3 : Constant  Value=1e-6  OutDataTypeStr=single  mask(TL_Constant){data={'output',{'type','Float32'},'date',735300.29224403936}}
      settings: CopyFcn=if exist('tl_reset_reviewflag','file')==2,tl_reset_reviewflag(gcbh);end  DeleteFcn=if exist('delete_tlblock','file')==2,delete_tlblock(gcbh);end  NameChangeFcn=if exist('rename_tlblock','file')==2,rename_tlblock(gcbh);end  OpenFcn=if exist('tl_open_blockdlg','file')==2,tl_open_blockdlg(gcbh);else,open_system(gcbh,'parameter');end
      mask Help: eval(['if exist(''tl_online_help'',''file'') == 2, tl_online_help(''Topic'',''TL_Constant''),else, web([''jar:file:///'',matlabroot,''/help/toolbox/simulink/help.jar!/slref/' lower(get_param(gcbh,'Blocktype')) '.html''], ''-helpbrowser''),end'])
      mask Display: plot([-0.05, 1.05, NaN, -0.05, 1.05],[.01, .01, NaN, .99, .99])
  Product : Product
  Product1 : Product
  Safe_Divide : Subsystem  mask(GL_SafeDivide_1.0){}
      mask help:
      | Safe Divide, prevents division by zero.
      |
      | if abs(denominator) > eps then
      |     output = numerator / denominator
      | else
      |     output = numerator / eps
      |
      | Attention!
      | Use this block only when there is a risk for division by zero.
      mask init:
      | set_param(gcb,'LinkStatus','none');
      mask Display:
      | port_label('input', 1, 'x')
      | port_label('input', 2, '÷')
      | port_label('input', 3, 'eps')
  Saturation : Subsystem  mask(GL_Saturation_1.0){}
      mask help:
      | If input_1 > input_2
      |   output = input_2
      | elseif input_1 < input_3
      |   output = input_3
      | else
      |   output = input_1
      |
      | Note that if the lower limit is set above the upper limit, the output will take the value of the input to the lower limit port.
      mask init:
      | set_param(gcb,'LinkStatus','none');
      mask Display: plot([0.3, 0.5, 0.7, 0.9], [0, 0, 1, 1])
  Out1 : Outport
  wires:
  x2/1 -> Add1/1
  Safe_Divide/1(Out1) -> Saturation/1(u)
  y2/1 -> Product1/2
  y1/1 -> Product/1
  Add3/1 -> Out1/1
  Add1/1 -> Safe_Divide/2(In2)
  Product/1 -> Add3/1
  Product1/1 -> Add3/2
  Add2/1 -> Product/2
  Saturation/1(y) -> Product1/1, Add2/2
  Constant2/1 -> Add2/1
  Constant1/1 -> Saturation/3(L)
  Constant/1 -> Saturation/2(U)
  Add/1 -> Safe_Divide/1(In3)
  x1/1 -> Add1/2, Add/2
  In1/1 -> Add/1
  One3/1 -> Safe_Divide/3(In1)

== system PCMULib/Standard/Math/Round ==
  In1 : Inport
  Add : Sum
  Add1 : Sum  Inputs=+-
  Constant : Constant  Value=0.5
  Constant1 : Constant
  mod : Subsystem  mask(PAG_mod_LV1.5_BV1){}
      mask help: Signed remainder after division.
      mask Display: disp('mod')
  Out1 : Outport
  wires:
  mod/1(Out1) -> Add1/2
  In1/1 -> Add/1
  Add/1 -> Add1/1, mod/1(In1)
  Add1/1 -> Out1/1
  Constant1/1 -> mod/2(In2)
  Constant/1 -> Add/2

== system PCMULib/Standard/Math/Safe_Divide ==
  In2 : Inport
  In1 : Inport  Port=2
  In3 : Inport  Port=3
  Constant : Constant  Value=0  OutDataTypeStr=Inherit: Inherit via back propagation
  Gain : Gain  Gain=-1
  LogicalSwitch : Subsystem  mask(PAG_Switch_LV1.6_BV2){}
      mask help:
      | Pass through input 1 when input 3 is true;
      | otherwise, pass through input 2
      mask Display:
      | plot([-0.1 0.2 0.2], [0.85 0.85 0.75])
      | plot([-0.1 0.2 0.2], [0.5 0.5 0.6])
      | plot([0.8 1.1], [0.5 0.5])
      | plot([0.15 0.8], [0.6 0.5])
      | plot([-0.1 0.5 0.5], [0.15 0.15 0.6])
  Max : MinMax  Function=max  Inputs=2
  MinMax1 : MinMax  Inputs=2
  Product1 : Product  Inputs=*/
  Relational Operator : RelationalOperator  Operator=<  OutDataTypeStr=boolean  InputSameDT=off
  Out1 : Outport
  wires:
  Relational Operator/1 -> LogicalSwitch/3(In3)
  Gain/1 -> MinMax1/2
  Product1/1 -> Out1/1
  Constant/1 -> Relational Operator/2
  In2/1 -> Product1/1
  LogicalSwitch/1(Out1) -> Product1/2
  Max/1 -> LogicalSwitch/2(In2)
  MinMax1/1 -> LogicalSwitch/1(In1)
  In3/1 -> Max/1, Gain/1
  In1/1 -> MinMax1/1, Max/2, Relational Operator/1

== system PCMULib/Standard/Math/Saturation ==
  u : Inport
  U : Inport  Port=2
  L : Inport  Port=3
  MinMax : MinMax  Inputs=2
  MinMax1 : MinMax  Function=max  Inputs=2
  y : Outport
  wires:
  MinMax/1 -> MinMax1/1
  U/1 -> MinMax/1
  u/1 -> MinMax/2
  MinMax1/1 -> y/1
  L/1 -> MinMax1/2

== system PCMULib/Standard/Math/mod ==
  In1 : Inport
  In2 : Inport  Port=2
  Mod : Math  Operator=mod  SignedPower=on
  Out1 : Outport
  wires:
  In1/1 -> Mod/1
  Mod/1 -> Out1/1
  In2/1 -> Mod/2

== system PCMULib/Standard/Math/rem ==
  In1 : Inport
  In2 : Inport  Port=2
  rem : Math  Operator=rem  SignedPower=on
  Out1 : Outport
  wires:
  In1/1 -> rem/1
  rem/1 -> Out1/1
  In2/1 -> rem/2

== system PCMULib/Standard/Math/sign_real ==
  In1 : Inport
  Constant : Constant  Value=-1
      settings: CopyFcn=set_param(gcbh,'ShowName','off');
  Constant1 : Constant
      settings: CopyFcn=set_param(gcbh,'ShowName','off');
  Constant2 : Constant  Value=0
      settings: CopyFcn=set_param(gcbh,'ShowName','off');
  Constant3 : Constant  Value=0
      settings: CopyFcn=set_param(gcbh,'ShowName','off');
  Constant4 : Constant  Value=0
      settings: CopyFcn=set_param(gcbh,'ShowName','off');
  Relational Operator : RelationalOperator  Operator===  OutDataTypeStr=boolean  InputSameDT=off
  Relational Operator1 : RelationalOperator  Operator=>  OutDataTypeStr=boolean  InputSameDT=off
  Switch : Switch  Criteria=u2 ~= 0  OutDataTypeStr=Inherit: Inherit via back propagation  RndMeth=Round
      mask init:
      | set_param(gcb,'LinkStatus','none');
      settings: CopyFcn=set_param(gcb,'showname','off');
      mask Display:
      | plot([0.54 0.65],[0.92 0.92])
      | plot([0.6 0.6],[0.84 0.92])
      | 
      | plot([0.54 0.54],[0.01 0.14])
      | plot([0.54 0.65],[0.14 0.14])
      | plot([0.54 0.625],[0.08 0.08])
  Switch1 : Switch  Criteria=u2 ~= 0  OutDataTypeStr=Inherit: Inherit via back propagation  RndMeth=Round
      mask init:
      | set_param(gcb,'LinkStatus','none');
      settings: CopyFcn=set_param(gcb,'showname','off');
      mask Display:
      | plot([0.54 0.65],[0.92 0.92])
      | plot([0.6 0.6],[0.84 0.92])
      | 
      | plot([0.54 0.54],[0.02 0.14])
      | plot([0.54 0.65],[0.14 0.14])
      | plot([0.54 0.625],[0.08 0.08])
  Out1 : Outport
  wires:
  Relational Operator/1 -> Switch1/2
  Relational Operator1/1 -> Switch/2
  Switch/1 -> Switch1/3
  Constant/1 -> Switch/3
  Constant1/1 -> Switch/1
  Constant2/1 -> Switch1/1
  Constant3/1 -> Relational Operator/2
  Constant4/1 -> Relational Operator1/2
  In1/1 -> Relational Operator1/1, Relational Operator/1
  Switch1/1 -> Out1/1

== system PCMULib/Standard/Math/xbackground1 ==

== system PCMULib/Standard/Math/xbackground10 ==

== system PCMULib/Standard/Math/xbackground2 ==

== system PCMULib/Standard/Math/xbackground3 ==

== system PCMULib/Standard/Relation&Logic/ConditionArbitration ==
  Condition1 : Inport  OutDataTypeStr=boolean
  Condition2 : Inport  Port=2  OutDataTypeStr=boolean
  Val_0_0 : Inport  Port=3
  Val_0_1 : Inport  Port=4
  Val_1_0 : Inport  Port=5
  Val_1_1 : Inport  Port=6
  Data Type Conversion : DataTypeConversion  RndMeth=Simplest
  Switch : Switch  Criteria=u2 ~= 0  OutDataTypeStr=Inherit: Inherit via back propagation  RndMeth=Simplest
      mask init:
      | set_param(gcb, 'LinkStatus', 'none');
      mask Display:
      | plot([0.54 0.65],[0.92 0.92])
      | plot([0.6 0.6],[0.84 0.92])
      | 
      | plot([0.54 0.54],[0.05 0.14])
      | plot([0.54 0.65],[0.14 0.14])
      | plot([0.54 0.625],[0.08 0.08])
  Switch1 : Switch  Criteria=u2 ~= 0  OutDataTypeStr=Inherit: Inherit via back propagation  RndMeth=Simplest
      mask init:
      | set_param(gcb, 'LinkStatus', 'none');
      mask Display:
      | plot([0.54 0.65],[0.92 0.92])
      | plot([0.6 0.6],[0.84 0.92])
      | 
      | plot([0.54 0.54],[0.05 0.14])
      | plot([0.54 0.65],[0.14 0.14])
      | plot([0.54 0.625],[0.08 0.08])
  Switch2 : Switch  Criteria=u2 ~= 0  OutDataTypeStr=Inherit: Inherit via back propagation  RndMeth=Simplest
      mask init:
      | set_param(gcb, 'LinkStatus', 'none');
      mask Display:
      | plot([0.54 0.65],[0.92 0.92])
      | plot([0.6 0.6],[0.84 0.92])
      | 
      | plot([0.54 0.54],[0.05 0.14])
      | plot([0.54 0.65],[0.14 0.14])
      | plot([0.54 0.625],[0.08 0.08])
  out : Outport
  wires:
  Data Type Conversion/1 -> out/1
  Switch1/1 -> Data Type Conversion/1
  Switch2/1 -> Switch1/3
  Val_0_1/1 -> Switch2/1
  Val_0_0/1 -> Switch2/3
  Val_1_0/1 -> Switch/3
  Switch/1 -> Switch1/1
  Val_1_1/1 -> Switch/1
  Condition1/1 -> Switch1/2
  Condition2/1 -> Switch/2, Switch2/2

== system PCMULib/Standard/Relation&Logic/CounterReset_dec ==
  e : Inport
  r : Inport  Port=2
  rv : Inport  Port=3
  dec : Inport  Port=4
  Add : Sum  Inputs=-+
  Constant : Constant  Value=0
  Constant1 : Constant  Value=0
  MinMax : MinMax  Function=max  Inputs=2
  Switch : Switch  Criteria=u2 ~= 0  Threshold=0.5  SaturateOnIntegerOverflow=off  InputSameDT=off
  Switch1 : Switch  Criteria=u2 ~= 0  Threshold=0.5  SaturateOnIntegerOverflow=off  InputSameDT=off
  Unit Delay : UnitDelay  SampleTime=-1  HasFrameUpgradeWarning=on
  y : Outport
  wires:
  Switch1/1 -> Add/1
  Constant1/1 -> Switch1/3
  dec/1 -> Switch1/1
  e/1 -> Switch1/2
  r/1 -> Switch/2
  Add/1 -> Switch/3
  rv/1 -> Switch/1
  Switch/1 -> MinMax/2
  Constant/1 -> MinMax/1
  MinMax/1 -> Unit Delay/1, y/1
  Unit Delay/1 -> Add/2

== system PCMULib/Standard/Relation&Logic/CounterReset_uint8 ==
  r : Inport
  rv : Inport  Port=2
  inc : Inport  Port=3
  Add : Sum  SaturateOnIntegerOverflow=on
  Switch1 : Switch  Criteria=u2 ~= 0  OutDataTypeStr=Inherit: Inherit via back propagation  RndMeth=Round
      mask init:
      | set_param(gcb,'LinkStatus','none');
      | % 这句的使用场景：
      | % 当模型没有这句时，模型传递给没有模型库的人员会出现红色的错误框
      | % 没有模型库的使用者不能查看此模块
      settings: CopyFcn=set_param(gcb,'showname','off');
      mask Display:
      | plot([0.54 0.65],[0.92 0.92])
      | plot([0.6 0.6],[0.84 0.92])
      | 
      | plot([0.54 0.54],[0.02 0.14])
      | plot([0.54 0.65],[0.14 0.14])
      | plot([0.54 0.625],[0.08 0.08])
  Unit Delay : UnitDelay  SampleTime=-1  HasFrameUpgradeWarning=on
  y : Outport
  wires:
  r/1 -> Switch1/2
  Add/1 -> Switch1/3
  rv/1 -> Switch1/1
  Unit Delay/1 -> Add/2
  inc/1 -> Add/1
  Switch1/1 -> y/1, Unit Delay/1

== system PCMULib/Standard/Relation&Logic/CounterReset_uint8_enable ==
  e : Inport
  r : Inport  Port=2
  rv : Inport  Port=3
  inc : Inport  Port=4
  Add : Sum  SaturateOnIntegerOverflow=on
  Constant1 : Constant  Value=0
  Switch : Switch  Criteria=u2 ~= 0  OutDataTypeStr=Inherit: Inherit via back propagation  RndMeth=Round
      mask init:
      | set_param(gcb,'LinkStatus','none');
      settings: CopyFcn=set_param(gcb,'showname','off');
      mask Display:
      | plot([0.54 0.65],[0.92 0.92])
      | plot([0.6 0.6],[0.84 0.92])
      | 
      | plot([0.54 0.54],[0.02 0.14])
      | plot([0.54 0.65],[0.14 0.14])
      | plot([0.54 0.625],[0.08 0.08])
  Switch1 : Switch  Criteria=u2 ~= 0  Threshold=0.5  SaturateOnIntegerOverflow=off  InputSameDT=off
  Unit Delay : UnitDelay  SampleTime=-1  HasFrameUpgradeWarning=on
  y : Outport
  wires:
  Unit Delay/1 -> Add/2
  rv/1 -> Switch/1
  Add/1 -> Switch/3
  r/1 -> Switch/2
  e/1 -> Switch1/2
  inc/1 -> Switch1/1
  Switch1/1 -> Add/1
  Constant1/1 -> Switch1/3
  Switch/1 -> y/1, Unit Delay/1

== system PCMULib/Standard/Relation&Logic/EdgeBi ==
  u : Inport
  AND : Logic  Operator=XOR  AllPortsSameDT=off  OutDataTypeStr=boolean
  Unit Delay : UnitDelay  SampleTime=-1  HasFrameUpgradeWarning=on
  y : Outport
  wires:
  AND/1 -> y/1
  Unit Delay/1 -> AND/2
  u/1 -> AND/1, Unit Delay/1

== system PCMULib/Standard/Relation&Logic/EdgeFalling ==
  In1 : Inport
  AND : Logic  Operator=NOT  Inputs=1  AllPortsSameDT=off  OutDataTypeStr=boolean
  AND1 : Logic  AllPortsSameDT=off  OutDataTypeStr=boolean
  Unit Delay : UnitDelay  SampleTime=-1  HasFrameUpgradeWarning=on
  Out1 : Outport
  wires:
  In1/1 -> AND/1, Unit Delay/1
  AND1/1 -> Out1/1
  Unit Delay/1 -> AND1/2
  AND/1 -> AND1/1

== system PCMULib/Standard/Relation&Logic/EdgeRising ==
  u : Inport
  AND : Logic  Operator=NOT  Inputs=1  AllPortsSameDT=off  OutDataTypeStr=boolean
  AND1 : Logic  AllPortsSameDT=off  OutDataTypeStr=boolean
  Unit Delay : UnitDelay  SampleTime=-1  HasFrameUpgradeWarning=on
  y : Outport
  wires:
  u/1 -> Unit Delay/1, AND1/1
  AND1/1 -> y/1
  Unit Delay/1 -> AND/1
  AND/1 -> AND1/2

== system PCMULib/Standard/Relation&Logic/If Action Subsystem ==
  In1 : Inport
  Action Port : ActionPort
  Out1 : Outport
  wires:
  In1/1 -> Out1/1

== system PCMULib/Standard/Relation&Logic/If-Then-Else ==
  If : Inport
  Then : Inport  Port=2
  Else : Inport  Port=3
  Switch : Switch  Criteria=u2 ~= 0  SaturateOnIntegerOverflow=off
      settings: AttributesFormatString=Require same data type on all input ports = %<InputSameDT>
  Out : Outport
  wires:
  Else/1 -> Switch/3
  Then/1 -> Switch/1
  If/1 -> Switch/2
  Switch/1 -> Out/1
